simulink model "PSAU_LV9"  (Simulink 7.8)
settings: Solver=ode45  StartTime=0.0  StopTime=500  RelTol=1e-3
values from neighbouring files (symbols this model uses):
  A1 = [-1/8 1/8 0 0; 0 -1/10 1/10 0;0 0 -1/1.2 1/1.2; 0 0 0 -1/0.8]    [Parametri.m]
  B1 = [0; 0; 0; 1/0.8]    [Parametri.m]
  C1 = [1 0 0 0]    [Parametri.m]
  D = 0    [Parametri.m]
  P1 = 0    [Parametri.m]
  Q1 = 1*eye(4,4)    [Parametri.m]
  R1 = 1    [Parametri.m]
  x10 = [0; 0; 0 ;0]    [Parametri.m]
libraries: simulink x2
settings Model: Creator=SUser  LastModifiedBy=AA
settings DebuggingCC: FcnCallInpInsideContextMsg=Use local settings

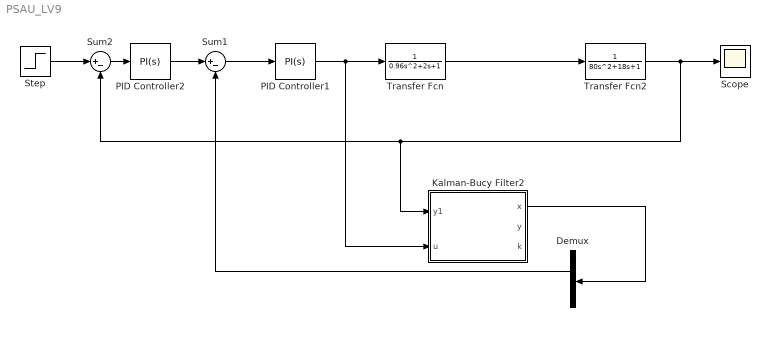
== system PSAU_LV9 ==
  Demux : Demux
  Kalman-Bucy Filter2 : Subsystem  mask{x0=x10, P0=P1, A=A1, B=B1, C=C1, D=D, Q=Q1, R=R1}
      mask Display:
      | port_label('input',1,'y')
      | port_label('input',2,'u')
      | port_label('output',1,'x')
      | port_label('output',2,'y')
      | disp(sprintf('Kalman-Bucy\n Filter'))
  PID Controller1 : simulink/Continuous/PID Controller  Controller=PI  TimeDomain=Continuous-time  SampleTime=1  IntegratorMethod=Forward Euler  FilterMethod=Forward Euler  Form=Parallel  P=1.76776695296637  I=1.04166666666667  D=-1612.79031123879  N=0.000390790797399611  InitialConditionSource=internal  InitialConditionForIntegrator=0  InitialConditionForFilter=0  ExternalReset=none  LimitOutput=off  UpperSaturationLimit=inf  LowerSaturationLimit=-inf  LinearizeAsGain=off  AntiWindupMode=none  Kb=1  TrackingMode=off  Kt=1  PParamMin=[]  PParamMax=[]  IParamMin=[]  IParamMax=[]  DParamMin=[]  DParamMax=[]  NParamMin=[]  NParamMax=[]  KbParamMin=[]  KbParamMax=[]  KtParamMin=[]  KtParamMax=[]  POutMin=[]  POutMax=[]  IOutMin=[]  IOutMax=[]  DOutMin=[]  DOutMax=[]  NOutMin=[]  NOutMax=[]  KbOutMin=[]  KbOutMax=[]  KtOutMin=[]  KtOutMax=[]  IntegratorOutMin=[]  IntegratorOutMax=[]  FilterOutMin=[]  FilterOutMax=[]  SumOutMin=[]  SumOutMax=[]  SumI1OutMin=[]  SumI1OutMax=[]  SumI2OutMin=[]  SumI2OutMax=[]  SumI3OutMin=[]  SumI3OutMax=[]  SumDOutMin=[]  SumDOutMax=[]  SaturationOutMin=[]  SaturationOutMax=[]  IntegratorContinuousStateAttributes=''  IntegratorStateMustResolveToSignalObject=off  IntegratorRTWStateStorageClass=Auto  FilterContinuousStateAttributes=''  FilterStateMustResolveToSignalObject=off  FilterRTWStateStorageClass=Auto
  PID Controller2 : simulink/Continuous/PID Controller  Controller=PI  TimeDomain=Continuous-time  SampleTime=1  IntegratorMethod=Forward Euler  FilterMethod=Forward Euler  Form=Parallel  P=0  I=0.0358919524069667  D=0  N=100  InitialConditionSource=internal  InitialConditionForIntegrator=0  InitialConditionForFilter=0  ExternalReset=none  LimitOutput=off  UpperSaturationLimit=inf  LowerSaturationLimit=-inf  LinearizeAsGain=off  AntiWindupMode=none  Kb=1  TrackingMode=off  Kt=1  PParamMin=[]  PParamMax=[]  IParamMin=[]  IParamMax=[]  DParamMin=[]  DParamMax=[]  NParamMin=[]  NParamMax=[]  KbParamMin=[]  KbParamMax=[]  KtParamMin=[]  KtParamMax=[]  POutMin=[]  POutMax=[]  IOutMin=[]  IOutMax=[]  DOutMin=[]  DOutMax=[]  NOutMin=[]  NOutMax=[]  KbOutMin=[]  KbOutMax=[]  KtOutMin=[]  KtOutMax=[]  IntegratorOutMin=[]  IntegratorOutMax=[]  FilterOutMin=[]  FilterOutMax=[]  SumOutMin=[]  SumOutMax=[]  SumI1OutMin=[]  SumI1OutMax=[]  SumI2OutMin=[]  SumI2OutMax=[]  SumI3OutMin=[]  SumI3OutMax=[]  SumDOutMin=[]  SumDOutMax=[]  SaturationOutMin=[]  SaturationOutMax=[]  IntegratorContinuousStateAttributes=''  IntegratorStateMustResolveToSignalObject=off  IntegratorRTWStateStorageClass=Auto  FilterContinuousStateAttributes=''  FilterStateMustResolveToSignalObject=off  FilterRTWStateStorageClass=Auto
  Scope : Scope
  Step : Step  Time=0  SampleTime=0
  Sum1 : Sum  Inputs=|+-
  Sum2 : Sum  Inputs=|+-
  Transfer Fcn : TransferFcn  Denominator=[0.96 2 1]
  Transfer Fcn2 : TransferFcn  Denominator=[80 18 1]
  wires:
  PID Controller1/1 -> Transfer Fcn/1, Kalman-Bucy Filter2/2(u)
  Transfer Fcn/1 -> Transfer Fcn2/1
  Sum1/1 -> PID Controller1/1
  Transfer Fcn2/1 -> Scope/1, Sum2/2, Kalman-Bucy Filter2/1(y1)
  PID Controller2/1 -> Sum1/1
  Step/1 -> Sum2/1
  Sum2/1 -> PID Controller2/1
  Demux/2 -> Sum1/2
  Kalman-Bucy Filter2/1(x) -> Demux/1

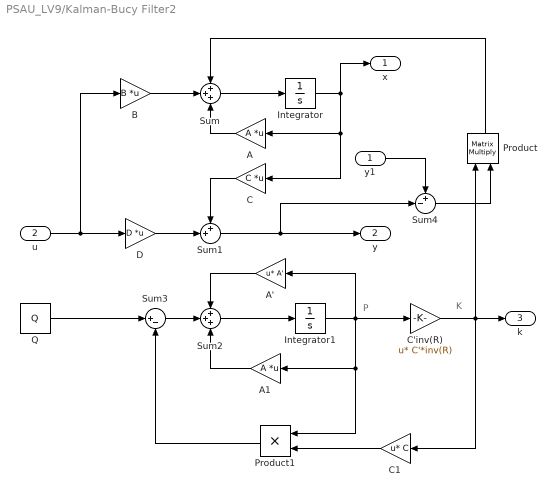
== system PSAU_LV9/Kalman-Bucy Filter2 ==
  note: K
  note: P
  y1 : Inport
  u : Inport  Port=2  PortDimensions=size(B,2)
  A : Gain  Gain=A  Multiplication=Matrix(K*u)
  A' : Gain  Gain=A'  Multiplication=Matrix(u*K)
  A1 : Gain  Gain=A  Multiplication=Matrix(K*u)
  B : Gain  Gain=B  Multiplication=Matrix(K*u)
  C : Gain  Gain=C  Multiplication=Matrix(K*u)
  C'inv(R) : Gain  Gain=C'*inv(R)  Multiplication=Matrix(u*K)
  C1 : Gain  Gain=C  Multiplication=Matrix(u*K)
  D : Gain  Gain=D  Multiplication=Matrix(K*u)
  Integrator : Integrator  InitialCondition=x0
  Integrator1 : Integrator  InitialCondition=P0
  Product : Product  Multiplication=Matrix(*)  RndMeth=Zero
  Product1 : Product  RndMeth=Zero
  Q : Constant  Value=Q
  Sum : Sum  Inputs=+++
  Sum1 : Sum  Inputs=++|
  Sum2 : Sum  Inputs=+++
  Sum3 : Sum  Inputs=|+-
  Sum4 : Sum  Inputs=+-|
  x : Outport
  y : Outport  Port=2
  k : Outport  Port=3
  wires:
  Sum1/1 -> y/1, Sum4/2
  D/1 -> Sum1/2
  C/1 -> Sum1/1
  B/1 -> Sum/2
  A/1 -> Sum/3
  Integrator/1 -> x/1, C/1, A/1
  Sum/1 -> Integrator/1
  u/1 -> D/1, B/1
  Sum2/1 -> Integrator1/1
  Integrator1/1 -> A'/1, C'inv(R)/1, A1/1, Product1/1
  A1/1 -> Sum2/3
  A'/1 -> Sum2/1
  Q/1 -> Sum3/1
  Sum3/1 -> Sum2/2
  y1/1 -> Sum4/1
  Product/1 -> Sum/1
  C'inv(R)/1 -> C1/1, Product/1, k/1
  Product1/1 -> Sum3/2
  C1/1 -> Product1/2
  Sum4/1 -> Product/2
